simulink model "longitudinal_tire"  (R2024b)
settings: Solver=VariableStepAuto  StartTime=0.0  StopTime=10  RelTol=1e-3
undefined symbols (not defined in the file): car
settings Model: Creator=Carlo  LastModifiedBy=franc
settings RTWCC: GPUComputeCapability=3.5

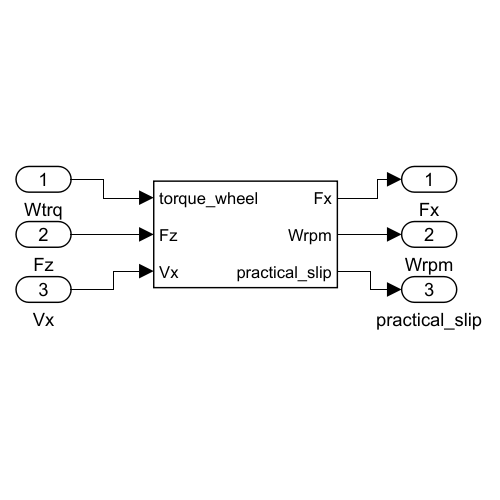
[thumbnail: Simulink's stored preview of the top-level diagram]
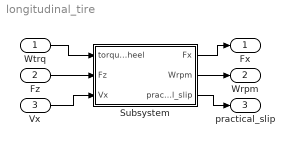
== system longitudinal_tire ==
  Wtrq : Inport
  Fz : Inport  Port=2
  Vx : Inport  Port=3
  Subsystem : Subsystem
  Fx : Outport
  Wrpm : Outport  Port=2
  practical_slip : Outport  Port=3
  wires:
  Wtrq/1 -> Subsystem/1(torque_wheel)
  Fz/1 -> Subsystem/2(Fz)
  Vx/1 -> Subsystem/3(Vx)
  Subsystem/1(Fx) -> Fx/1
  Subsystem/2(Wrpm) -> Wrpm/1
  Subsystem/3(practical_slip) -> practical_slip/1

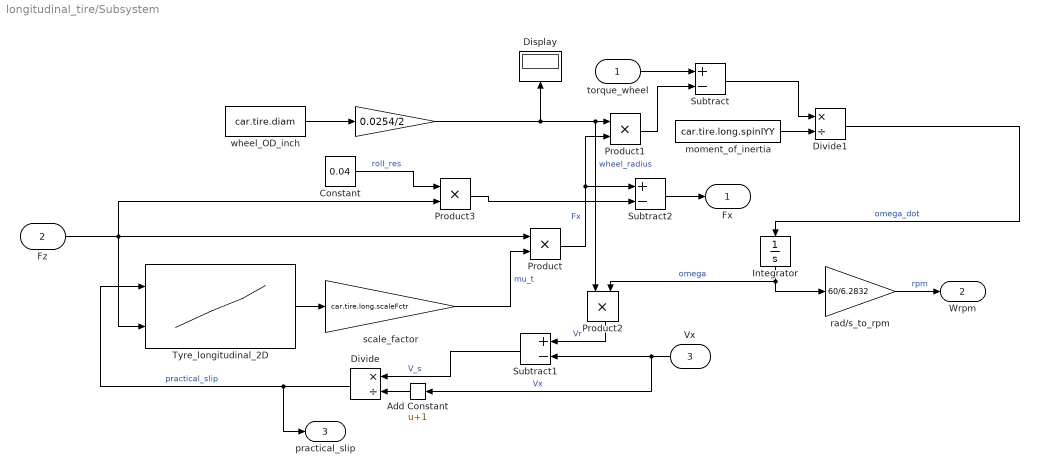
== system longitudinal_tire/Subsystem ==
  torque_wheel : Inport
  Fz : Inport  Port=2
  Vx : Inport  Port=3
  " " : Gain  Gain=0.0254/2
  Add Constant : Bias  Bias=1  SaturateOnIntegerOverflow=off
  Constant : Constant  Value=0.04
  Display : Display
  Divide : Product  Inputs=*/
  Divide1 : Product  Inputs=*/
  Integrator : Integrator
  Product{,1..3} (4 alike) : Product
  Subtract : Sum  Inputs=+-
  Subtract1 : Sum  Inputs=+-
  Subtract2 : Sum  Inputs=+-
  Tyre_longitudinal_2D : Lookup_n-D  BreakpointsForDimension1=[-1 -0.8 -0.4 -0.2 -0.1 0 0.1 0.2 0.4 0.8 1]  BreakpointsForDimension2=[340 540 740 940 1140]  Table=[-2.22 -2.18 -2.14 -2.11 -2.11;-2.21 -2.18 -2.15 -2.12 -2.12;-2.25 -2.21 -2.17 -2.15 -2.14;-2.27 -2.24 -2.21 -2.18 -2.07;-2.26 -2.2 -2.14 -2.01 -1.68;0 0 0 0 0;2.26 2.2 2.14 2.01 1.68;2.27 2.24 2.21 2.18 2.07;2.25 2.21 2.17 2.15 2.14;2.21 2.18 2.15 2.12 2.12;2.22 2.18 2.14 2.11 2.11]  InternalRulePriority=Speed  RndMeth=Simplest
      settings: InputPortMap=u0,u1
  moment_of_inertia : Constant  Value=car.tire.long.spinIYY
  rad/s_to_rpm : Gain  Gain=60/6.2832
  scale_factor : Gain  Gain=car.tire.long.scaleFctr
  wheel_OD_inch : Constant  Value=car.tire.diam
  Fx : Outport
  Wrpm : Outport  Port=2
  practical_slip : Outport  Port=3
  wires:
  Subtract/1 -> Divide1/1
  Product2/1 -> Subtract1/1  "Vr"
  Subtract1/1 -> Divide/1  "V_s"
  Product1/1 -> Subtract/2
  " "/1 -> Product1/1, Product2/1, Display/1  "wheel_radius"
  Fz/1 -> Product3/2, Product/1, Tyre_longitudinal_2D/2
  Divide1/1 -> Integrator/1  "omega_dot"
  wheel_OD_inch/1 -> " "/1
  Divide/1 -> practical_slip/1, Tyre_longitudinal_2D/1  "practical_slip"
  Product/1 -> Subtract2/1, Product1/2  "Fx"
  moment_of_inertia/1 -> Divide1/2
  Add Constant/1 -> Divide/2
  torque_wheel/1 -> Subtract/1
  Tyre_longitudinal_2D/1 -> scale_factor/1
  scale_factor/1 -> Product/2  "mu_t"
  Integrator/1 -> rad/s_to_rpm/1, Product2/2  "omega"
  rad/s_to_rpm/1 -> Wrpm/1  "rpm"
  Vx/1 -> Add Constant/1, Subtract1/2  "Vx"
  Constant/1 -> Product3/1  "roll_res"
  Subtract2/1 -> Fx/1
  Product3/1 -> Subtract2/2
